simulink model "PV_model"  (R2018a)
settings: Solver=VariableStepAuto  StartTime=0.0  StopTime=1  RelTol=1e-3
libraries: simulink x1
settings Model: Creator=DELL  LastModifiedBy=DELL

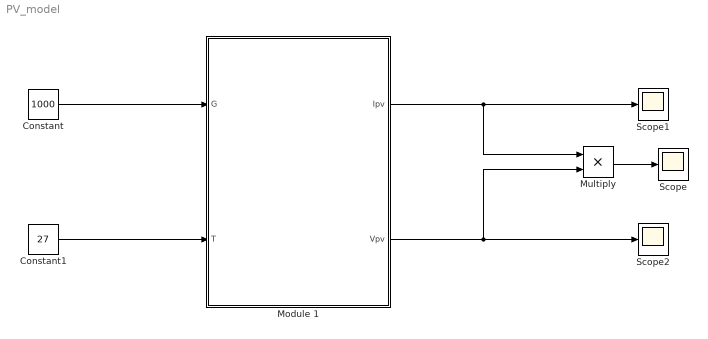
== system PV_model ==
  Constant : Constant  Value=1000
  Constant1 : Constant  Value=27
  "Module 1 " : Subsystem
  Multiply : Product
  Scope : Scope
  Scope1 : Scope
  Scope2 : Scope
  wires:
  Constant1/1 -> "Module 1 "/2(T)
  Constant/1 -> "Module 1 "/1(G)
  "Module 1 "/1(Ipv) -> Scope1/1, Multiply/1
  "Module 1 "/2("Vpv ") -> Scope2/1, Multiply/2
  Multiply/1 -> Scope/1

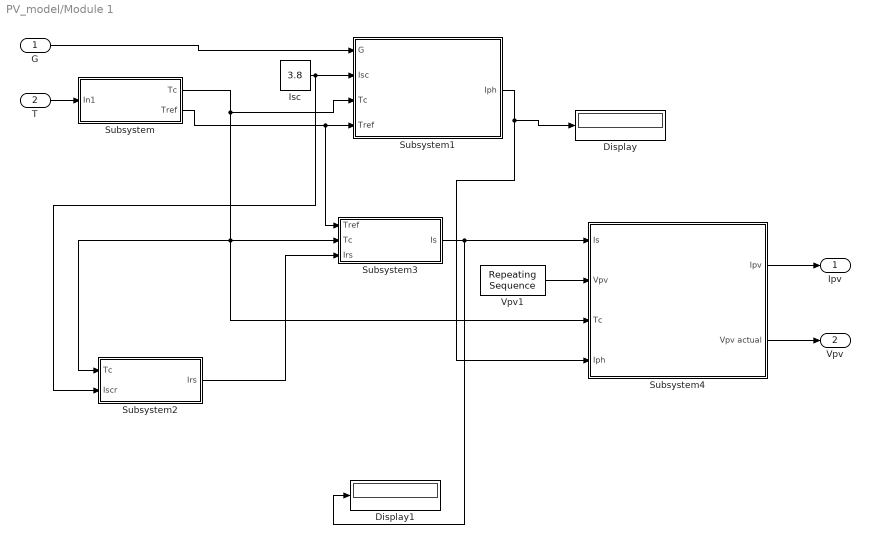
== system PV_model/Module 1  ==
  G : Inport
  T : Inport  Port=2
  Display : Display
  Display1 : Display
  "Isc " : Constant  Value=3.8
  Subsystem : Subsystem
  Subsystem1 : Subsystem
  Subsystem2 : Subsystem
  Subsystem3 : Subsystem
  Subsystem4 : Subsystem
  Vpv1 : simulink/Sources/Repeating Sequence  rep_seq_t=[0 1 2]  rep_seq_y=[0 21 0]
  Ipv : Outport
  "Vpv " : Outport  Port=2
  wires:
  "Isc "/1 -> Subsystem2/2(Iscr), Subsystem1/2(Isc)
  Subsystem/1(Tc) -> Subsystem4/3(Tc), Subsystem2/1(Tc), Subsystem3/2(Tc), Subsystem1/3(Tc)
  Subsystem/2("Tref ") -> Subsystem3/1(Tref), Subsystem1/4(Tref)
  G/1 -> Subsystem1/1(G)
  Subsystem2/1(Irs) -> Subsystem3/3("Irs ")
  Subsystem1/1(Iph) -> Display/1, Subsystem4/4("Iph ")
  Vpv1/1 -> Subsystem4/2(Vpv)
  Subsystem3/1(Is) -> Display1/1, Subsystem4/1("Is ")
  T/1 -> Subsystem/1(In1)
  Subsystem4/1(Ipv) -> Ipv/1
  Subsystem4/2(Vpv actual) -> "Vpv "/1

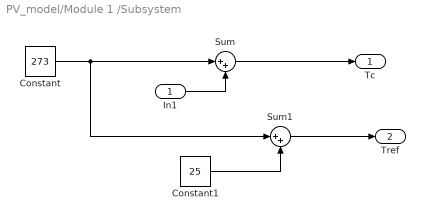
== system PV_model/Module 1 /Subsystem ==
  In1 : Inport
  Constant : Constant  Value=273
  Constant1 : Constant  Value=25
  Sum : Sum  Inputs=|++
  Sum1 : Sum  Inputs=|++
  Tc : Outport
  "Tref " : Outport  Port=2
  wires:
  In1/1 -> Sum/2
  Constant/1 -> Sum/1, Sum1/1
  Constant1/1 -> Sum1/2
  Sum/1 -> Tc/1
  Sum1/1 -> "Tref "/1

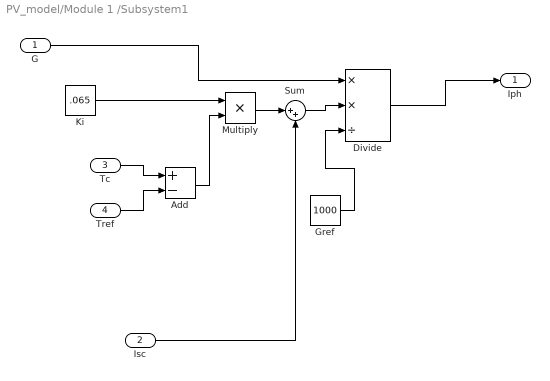
== system PV_model/Module 1 /Subsystem1 ==
  G : Inport
  Isc : Inport  Port=2
  Tc : Inport  Port=3
  Tref : Inport  Port=4
  Add : Sum  Inputs=+-
  Divide : Product  Inputs=**/
  Gref : Constant  Value=1000
  Ki : Constant  Value=.065
  Multiply : Product
  Sum : Sum  Inputs=|++
  Iph : Outport
  wires:
  Tc/1 -> Add/1
  Tref/1 -> Add/2
  Add/1 -> Multiply/2
  Ki/1 -> Multiply/1
  Multiply/1 -> Sum/1
  Isc/1 -> Sum/2
  G/1 -> Divide/1
  Sum/1 -> Divide/2
  Gref/1 -> Divide/3
  Divide/1 -> Iph/1

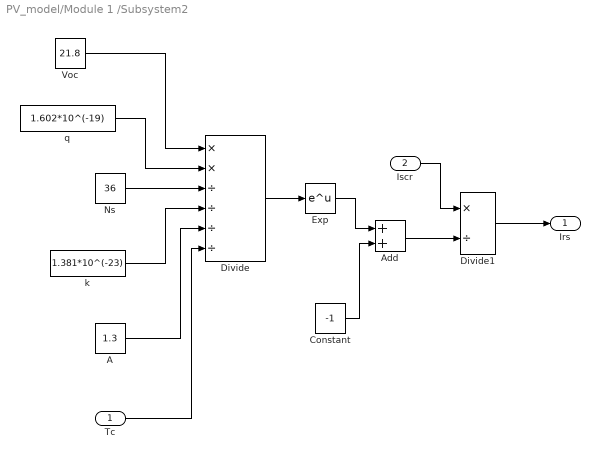
== system PV_model/Module 1 /Subsystem2 ==
  Tc : Inport
  Iscr : Inport  Port=2
  A : Constant  Value=1.3
  Add : Sum
  Constant : Constant  Value=-1
  Divide : Product  Inputs=**////
  Divide1 : Product  Inputs=*/
  Exp : Math  SaturateOnIntegerOverflow=on
  Ns : Constant  Value=36
  "Voc " : Constant  Value=21.8
  k : Constant  Value=1.381*10^(-23)
  q : Constant  Value=1.602*10^(-19)
  Irs : Outport
  wires:
  "Voc "/1 -> Divide/1
  q/1 -> Divide/2
  Ns/1 -> Divide/3
  k/1 -> Divide/4
  A/1 -> Divide/5
  Tc/1 -> Divide/6
  Divide/1 -> Exp/1
  Exp/1 -> Add/1
  Constant/1 -> Add/2
  Add/1 -> Divide1/2
  Iscr/1 -> Divide1/1
  Divide1/1 -> Irs/1

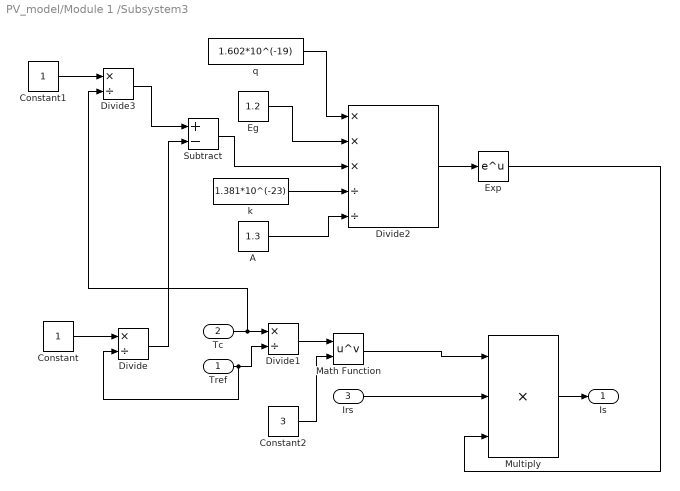
== system PV_model/Module 1 /Subsystem3 ==
  Tref : Inport
  Tc : Inport  Port=2
  "Irs " : Inport  Port=3
  A : Constant  Value=1.3
  Constant : Constant
  Constant1 : Constant
  Constant2 : Constant  Value=3
  Divide : Product  Inputs=*/
  Divide1 : Product  Inputs=*/
  Divide2 : Product  Inputs=***//
  Divide3 : Product  Inputs=*/
  Eg : Constant  Value=1.2
  Exp : Math  SaturateOnIntegerOverflow=on
  Math Function : Math  Operator=pow  SaturateOnIntegerOverflow=on
  Multiply : Product  Inputs=3
  Subtract : Sum  Inputs=+-
  k : Constant  Value=1.381*10^(-23)
  q : Constant  Value=1.602*10^(-19)
  Is : Outport
  wires:
  Constant/1 -> Divide/1
  Tref/1 -> Divide/2, Divide1/2
  Math Function/1 -> Multiply/1
  "Irs "/1 -> Multiply/2
  Multiply/1 -> Is/1
  Exp/1 -> Multiply/3
  Divide2/1 -> Exp/1
  k/1 -> Divide2/4
  A/1 -> Divide2/5
  Tc/1 -> Divide3/2, Divide1/1
  Constant1/1 -> Divide3/1
  Divide3/1 -> Subtract/1
  Divide/1 -> Subtract/2
  Subtract/1 -> Divide2/3
  Eg/1 -> Divide2/2
  q/1 -> Divide2/1
  Divide1/1 -> Math Function/1
  Constant2/1 -> Math Function/2

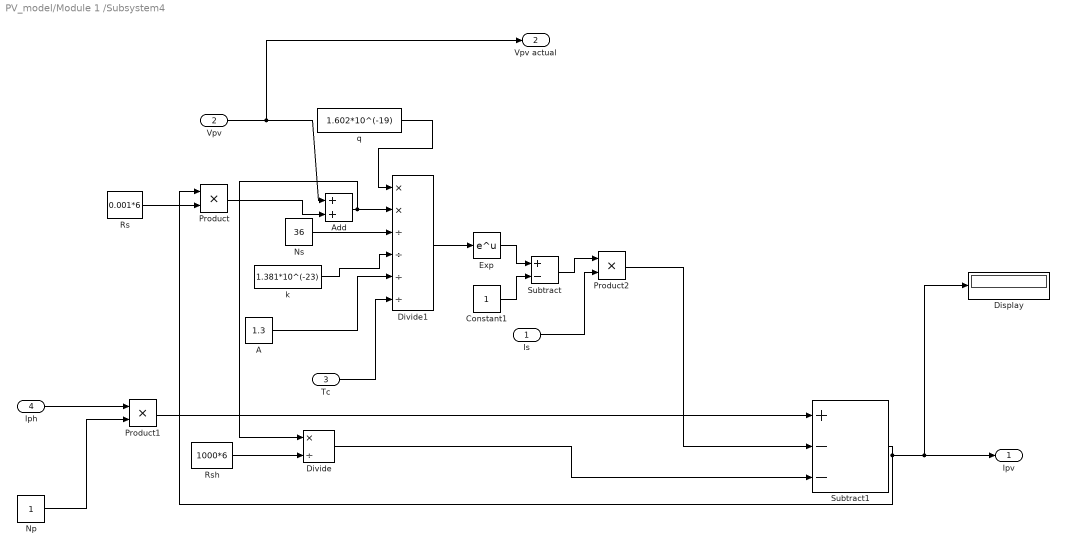
== system PV_model/Module 1 /Subsystem4 ==
  "Is " : Inport
  Vpv : Inport  Port=2
  Tc : Inport  Port=3
  "Iph " : Inport  Port=4
  A : Constant  Value=1.3
  Add : Sum
  Constant1 : Constant
  Display : Display
  Divide : Product  Inputs=*/
  Divide1 : Product  Inputs=**////
  Exp : Math  SaturateOnIntegerOverflow=on
  Np : Constant
  Ns : Constant  Value=36
  Product : Product
  Product1 : Product
  Product2 : Product
  Rs : Constant  Value=0.001*6
  Rsh : Constant  Value=1000*6
  Subtract : Sum  Inputs=+-
  Subtract1 : Sum  Inputs=+--
  k : Constant  Value=1.381*10^(-23)
  q : Constant  Value=1.602*10^(-19)
  Ipv : Outport
  Vpv actual : Outport  Port=2
  wires:
  Rsh/1 -> Divide/2
  k/1 -> Divide1/4
  A/1 -> Divide1/5
  Ns/1 -> Divide1/3
  Divide1/1 -> Exp/1
  Exp/1 -> Subtract/1
  Constant1/1 -> Subtract/2
  Subtract/1 -> Product2/1
  "Is "/1 -> Product2/2
  Product/1 -> Add/2
  Vpv/1 -> Vpv actual/1, Add/1
  Add/1 -> Divide/1, Divide1/2
  Tc/1 -> Divide1/6
  q/1 -> Divide1/1
  "Iph "/1 -> Product1/1
  Rs/1 -> Product/2
  Np/1 -> Product1/2
  Product1/1 -> Subtract1/1
  Product2/1 -> Subtract1/2
  Subtract1/1 -> Product/1, Display/1, Ipv/1
  Divide/1 -> Subtract1/3
